simulink model "vehicleVariantsLabel"  (R2020a)
settings: Solver=VariableStepAuto  StartTime=0.0  StopTime=30  FixedStep=Ts  RelTol=1e-3
model workspace: external: MAT-File data.mat (data not in the file)
values from neighbouring files (symbols this model uses):
  fsw = 9000    [data.mat]
  ID_MAP = [-123.486133396 -123.486133396 -123.486133396 -123.486133396 -123.486133396 -123.486133396 -123.486133396 -123.486133396 -123.486133396 -123.486133396 -123.486133396 -123.486133396 ... (280623 elements, 161x83x21)]    [data.mat]
  IQ_MAP = [-339.521551914 -339.521551914 -339.521551914 -339.521551914 -339.521551914 -339.521551914 -339.521551914 -339.521551914 -339.521551914 -339.521551914 -339.521551914 -339.521551914 ... (280623 elements, 161x83x21)]    [data.mat]
  Ki_v = 70    [data.mat]
  Kp_v = 150    [data.mat]
  Ld = 0.00024368    [data.mat]
  Lq = 0.00029758    [data.mat]
  motorOn = 1    [data.mat]
  p = 8    [data.mat]
  Pmax = 35000    [data.mat]
  psim = 0.04366    [data.mat]
  recumax = -50    [data.mat]
  RPM_VECT = [0 100 200 300 400 500 600 700 800 900 1000 1100 ... (161 elements, 1x161)]    [data.mat]
  rreifen = 0.3237    [data.mat]
  Tmax = 205    [data.mat]
  TQ_VECT = [-205 -200 -195 -190 -185 -180 -175 -170 -165 -160 -155 -150 ... (83 elements, 1x83)]    [data.mat]
  Ts = 5e-05    [data.mat]
  Tsi = 5e-05    [data.mat]
  Tso = 0.0005    [data.mat]
  VDC_VECT = [300 305 310 315 320 325 330 335 340 345 350 355 ... (21 elements, 1x21)]    [data.mat]
  Vnom = 325    [data.mat]
undefined symbols (not defined in the file or in its folder): DiscIntNeverNeededParam, sigbuilder_block
libraries: fl_lib x42, nesl_utility x20, ee_lib x8, simulink x2, eeTransforms x2, eeDiscretePi x1, eePmsmCurrentController x1, eePwmGeneratorTwoLevel x1
(part 2 of 2)

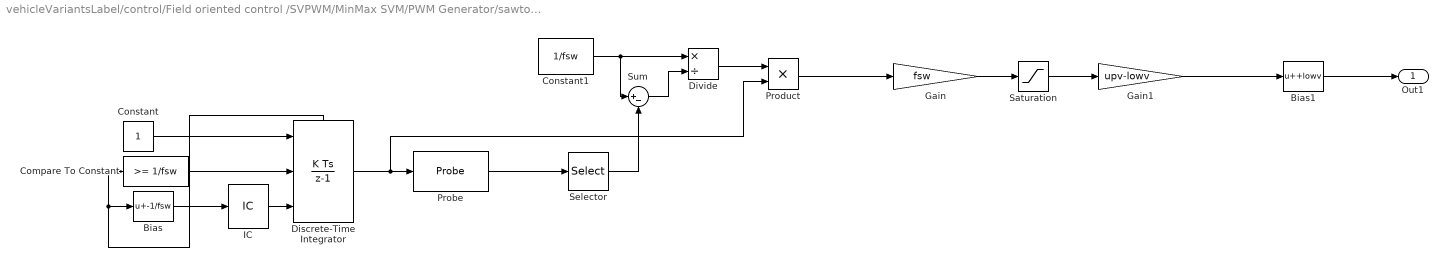
== system vehicleVariantsLabel/control/Field oriented control /SVPWM/MinMax SVM/PWM Generator/sawtooth ==
  Bias : Bias  Bias=-1/fsw
  Bias1 : Bias  Bias=+lowv
  Compare To Constant : simulink/Logic and Bit Operations/Compare To Constant  relop=>=  const=1/fsw  OutDataTypeStr=boolean
  Constant : Constant  SampleTime=-1
  Constant1 : Constant  Value=1/fsw  SampleTime=-1
  Discrete-Time Integrator : DiscreteIntegrator  ExternalReset=rising  InitialConditionSource=external  SampleTime=-1  ShowStatePort=on  ICPrevOutput=DiscIntNeverNeededParam  ICPrevScaledInput=DiscIntNeverNeededParam
  Divide : Product  Inputs=*/
  Gain : Gain  Gain=fsw
  Gain1 : Gain  Gain=upv-lowv
  IC : InitialCondition  Value=0
  Probe : Probe  ProbeWidth=off  ProbeComplexSignal=off
  Product : Product
  Saturation : Saturate  UpperLimit=1  LowerLimit=0
  Selector : Selector  InputPortWidth=2  IndexOptions=Index vector (dialog)  Indices=1  OutputSizes=1
  Sum : Sum  Inputs=|+-
  Out1 : Outport  VectorParamsAs1DForOutWhenUnconnected=off
  wires:
  Saturation/1 -> Gain1/1
  Gain1/1 -> Bias1/1
  Probe/1 -> Selector/1
  Sum/1 -> Divide/2
  Gain/1 -> Saturation/1
  Compare To Constant/1 -> Discrete-Time Integrator/2
  Discrete-Time Integrator/State -> Bias/1, Compare To Constant/1
  Bias/1 -> IC/1
  Constant/1 -> Discrete-Time Integrator/1
  IC/1 -> Discrete-Time Integrator/3
  Constant1/1 -> Divide/1, Sum/1
  Discrete-Time Integrator/1 -> Probe/1, Product/2
  Divide/1 -> Product/1
  Bias1/1 -> Out1/1
  Selector/1 -> Sum/2
  Product/1 -> Gain/1
